simulink model "PII_speed"  (Simulink 7.5)
settings: Solver=ode1  SolverMode=SingleTasking  StartTime=0.0  StopTime=Inf  FixedStep=ts  RelTol=1e-3
PostLoadFcn:
  | , if any(exist('dsrtsu_mdlpostloadfcn', 'file') == [2, 3, 6]), try dsrtsu_mdlpostloadfcn('Execute', bdroot); catch fprintf('Error in PostLoadFcn (dsrtsu_mdlpostloadfcn) for model "%s":\n %s\n', bdroot, lasterr); end, end,
values from neighbouring files (symbols this model uses):
  Amp = 0    [RUN.m]
  en = 0    [RUN.m]
  f = 0.20    (= 0.2)    [RUN.m]
  g = 1    [RUN.m]
  kii = 660    [RUN.m]
  kpi = 2.0    (= 2)    [RUN.m]
  limit = 1    [RUN.m]
  nap = 0    [RUN.m]
  obc_del = 0.7    [RUN.m]
  obc_del2 = 1.3    [RUN.m]
  obc_en = 0    [RUN.m]
  obc_en1 = 0    [RUN.m]
  offset = 0    [RUN.m]
  res = 1    [RUN.m]
  res1 = 1    [RUN.m]
  start = 0    [RUN.m]
  Tf = 0.01    [RUN.m]
  Ts_i = 0.0002    [RUN.m]
  Ts_w = 0.001    [RUN.m]
undefined symbols (not defined in the file or in its folder): k1_singletons, k1k, k2_singletons, k2k, k3_singletons, k3k, kdu, Ki_singletons, Kik, ku, mf
libraries: fuzblock x15, rtilib1103 x6, simulink_extras x1
(part 2 of 2)

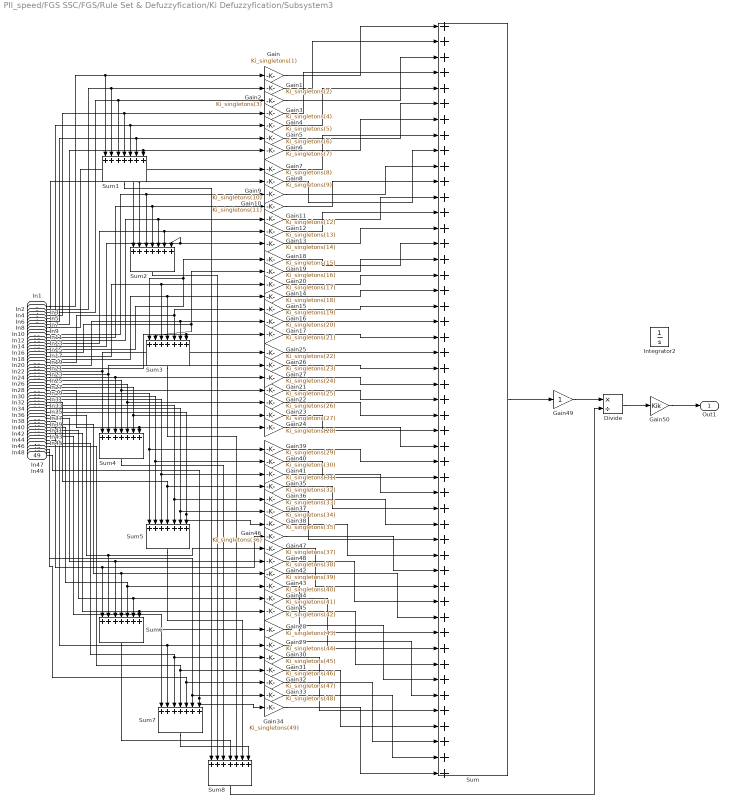
== system PII_speed/FGS SSC/FGS/Rule Set & Defuzzyfication/Ki Defuzzyfication/Subsystem3 ==
  In1 : Inport
  In2 : Inport  Port=2
  In3 : Inport  Port=3
  In4 : Inport  Port=4
  In5 : Inport  Port=5
  In6 : Inport  Port=6
  In7 : Inport  Port=7
  In8 : Inport  Port=8
  In9 : Inport  Port=9
  In10 : Inport  Port=10
  In11 : Inport  Port=11
  In12 : Inport  Port=12
  In13 : Inport  Port=13
  In14 : Inport  Port=14
  In15 : Inport  Port=15
  In16 : Inport  Port=16
  In17 : Inport  Port=17
  In18 : Inport  Port=18
  In19 : Inport  Port=19
  In20 : Inport  Port=20
  In21 : Inport  Port=21
  In22 : Inport  Port=22
  In23 : Inport  Port=23
  In24 : Inport  Port=24
  In25 : Inport  Port=25
  In26 : Inport  Port=26
  In27 : Inport  Port=27
  In28 : Inport  Port=28
  In29 : Inport  Port=29
  In30 : Inport  Port=30
  In31 : Inport  Port=31
  In32 : Inport  Port=32
  In33 : Inport  Port=33
  In34 : Inport  Port=34
  In35 : Inport  Port=35
  In36 : Inport  Port=36
  In37 : Inport  Port=37
  In38 : Inport  Port=38
  In39 : Inport  Port=39
  In40 : Inport  Port=40
  In41 : Inport  Port=41
  In42 : Inport  Port=42
  In43 : Inport  Port=43
  In44 : Inport  Port=44
  In45 : Inport  Port=45
  In46 : Inport  Port=46
  In47 : Inport  Port=47
  In48 : Inport  Port=48
  In49 : Inport  Port=49
  Divide : Product  Inputs=*/
  Gain : Gain  Gain=Ki_singletons(1)
  Gain1 : Gain  Gain=Ki_singletons(2)
  Gain10 : Gain  Gain=Ki_singletons(11)
  Gain11 : Gain  Gain=Ki_singletons(12)
  Gain12 : Gain  Gain=Ki_singletons(13)
  Gain13 : Gain  Gain=Ki_singletons(14)
  Gain14 : Gain  Gain=Ki_singletons(18)
  Gain15 : Gain  Gain=Ki_singletons(19)
  Gain16 : Gain  Gain=Ki_singletons(20)
  Gain17 : Gain  Gain=Ki_singletons(21)
  Gain18 : Gain  Gain=Ki_singletons(15)
  Gain19 : Gain  Gain=Ki_singletons(16)
  Gain2 : Gain  Gain=Ki_singletons(3)
  Gain20 : Gain  Gain=Ki_singletons(17)
  Gain21 : Gain  Gain=Ki_singletons(25)
  Gain22 : Gain  Gain=Ki_singletons(26)
  Gain23 : Gain  Gain=Ki_singletons(27)
  Gain24 : Gain  Gain=Ki_singletons(28)
  Gain25 : Gain  Gain=Ki_singletons(22)
  Gain26 : Gain  Gain=Ki_singletons(23)
  Gain27 : Gain  Gain=Ki_singletons(24)
  Gain28 : Gain  Gain=Ki_singletons(43)
  Gain29 : Gain  Gain=Ki_singletons(44)
  Gain3 : Gain  Gain=Ki_singletons(4)
  Gain30 : Gain  Gain=Ki_singletons(45)
  Gain31 : Gain  Gain=Ki_singletons(46)
  Gain32 : Gain  Gain=Ki_singletons(47)
  Gain33 : Gain  Gain=Ki_singletons(48)
  Gain34 : Gain  Gain=Ki_singletons(49)
  Gain35 : Gain  Gain=Ki_singletons(32)
  Gain36 : Gain  Gain=Ki_singletons(33)
  Gain37 : Gain  Gain=Ki_singletons(34)
  Gain38 : Gain  Gain=Ki_singletons(35)
  Gain39 : Gain  Gain=Ki_singletons(29)
  Gain4 : Gain  Gain=Ki_singletons(5)
  Gain40 : Gain  Gain=Ki_singletons(30)
  Gain41 : Gain  Gain=Ki_singletons(31)
  Gain42 : Gain  Gain=Ki_singletons(39)
  Gain43 : Gain  Gain=Ki_singletons(40)
  Gain44 : Gain  Gain=Ki_singletons(41)
  Gain45 : Gain  Gain=Ki_singletons(42)
  Gain46 : Gain  Gain=Ki_singletons(36)
  Gain47 : Gain  Gain=Ki_singletons(37)
  Gain48 : Gain  Gain=Ki_singletons(38)
  Gain49 : Gain
  Gain5 : Gain  Gain=Ki_singletons(6)
  Gain50 : Gain  Gain=Kik
  Gain6 : Gain  Gain=Ki_singletons(7)
  Gain7 : Gain  Gain=Ki_singletons(8)
  Gain8 : Gain  Gain=Ki_singletons(9)
  Gain9 : Gain  Gain=Ki_singletons(10)
  Integrator2 : Integrator
  Sum : Sum  Inputs=49
  Sum{1..8} (8 alike) : Sum  Inputs=7
  Out1 : Outport
  wires:
  Gain49/1 -> Divide/1
  In4/1 -> Sum1/4, Gain3/1
  Gain25/1 -> Sum/22
  Gain/1 -> Sum/1
  Gain34/1 -> Sum/49
  Gain39/1 -> Sum/29
  Gain13/1 -> Sum/14
  Gain17/1 -> Sum/21
  Gain19/1 -> Sum/16
  Gain12/1 -> Sum/13
  Gain40/1 -> Sum/30
  Gain35/1 -> Sum/32
  Gain9/1 -> Sum/10
  Gain6/1 -> Sum/7
  Gain27/1 -> Sum/24
  Gain11/1 -> Sum/12
  Gain15/1 -> Sum/19
  Gain10/1 -> Sum/11
  Gain22/1 -> Sum/26
  Gain23/1 -> Sum/27
  Gain8/1 -> Sum/9
  Gain38/1 -> Sum/35
  Gain46/1 -> Sum/36
  Gain37/1 -> Sum/34
  Gain16/1 -> Sum/20
  Gain36/1 -> Sum/33
  Gain18/1 -> Sum/15
  Gain14/1 -> Sum/18
  Gain5/1 -> Sum/6
  Gain47/1 -> Sum/37
  Gain26/1 -> Sum/23
  Gain4/1 -> Sum/5
  Gain7/1 -> Sum/8
  Gain20/1 -> Sum/17
  Gain41/1 -> Sum/31
  Gain21/1 -> Sum/25
  Gain24/1 -> Sum/28
  Sum2/1 -> Sum8/2
  Gain33/1 -> Sum/48
  Gain1/1 -> Sum/2
  Sum6/1 -> Sum8/4
  Sum5/1 -> Sum8/6
  Sum4/1 -> Sum8/3
  Sum/1 -> Gain49/1
  Sum8/1 -> Divide/2
  Gain31/1 -> Sum/46
  Gain3/1 -> Sum/4
  Gain44/1 -> Sum/41
  Gain28/1 -> Sum/43
  Gain42/1 -> Sum/39
  Gain2/1 -> Sum/3
  Sum7/1 -> Sum8/7
  Gain29/1 -> Sum/44
  Gain45/1 -> Sum/42
  Gain32/1 -> Sum/47
  Gain30/1 -> Sum/45
  Gain48/1 -> Sum/38
  Gain43/1 -> Sum/40
  Sum1/1 -> Sum8/1
  Sum3/1 -> Sum8/5
  In17/1 -> Sum3/3, Gain20/1
  In20/1 -> Sum3/6, Gain16/1
  In18/1 -> Sum3/4, Gain14/1
  In10/1 -> Sum2/3, Gain9/1
  In14/1 -> Sum2/7, Gain13/1
  In9/1 -> Sum2/2, Gain8/1
  In3/1 -> Sum1/3, Gain2/1
  In15/1 -> Gain18/1, Sum3/1
  In8/1 -> Sum2/1, Gain7/1
  In38/1 -> Gain46/1, Sum6/1
  In37/1 -> Gain48/1, Sum6/3
  In24/1 -> Sum4/3, Gain27/1
  In31/1 -> Gain41/1, Sum5/3
  In22/1 -> Gain25/1, Sum4/1
  In21/1 -> Sum3/7, Gain17/1
  In34/1 -> Gain37/1, Sum5/6
  In19/1 -> Gain15/1, Sum3/5
  In26/1 -> Sum4/5, Gain22/1
  In41/1 -> Gain44/1, Sum6/6
  In43/1 -> Gain28/1, Sum7/1
  In11/1 -> Sum2/4, Gain10/1
  In16/1 -> Gain19/1, Sum3/2
  In25/1 -> Sum4/4, Gain21/1
  In28/1 -> Sum4/7, Gain24/1
  In35/1 -> Gain38/1, Sum5/7
  In12/1 -> Sum2/5, Gain11/1
  In13/1 -> Sum2/6, Gain12/1
  In40/1 -> Gain43/1, Sum6/5
  In33/1 -> Gain36/1, Sum5/5
  In29/1 -> Gain39/1, Sum5/1
  In23/1 -> Gain26/1, Sum4/2
  In36/1 -> Gain47/1, Sum6/2
  In27/1 -> Sum4/6, Gain23/1
  In32/1 -> Gain35/1, Sum5/4
  In30/1 -> Gain40/1, Sum5/2
  In42/1 -> Gain45/1, Sum6/7
  In49/1 -> Gain34/1, Sum7/7
  In44/1 -> Sum7/2, Gain29/1
  In39/1 -> Gain42/1, Sum6/4
  In6/1 -> Sum1/6, Gain5/1
  In46/1 -> Gain31/1, Sum7/4
  In2/1 -> Sum1/2, Gain1/1
  In47/1 -> Gain32/1, Sum7/5
  In5/1 -> Sum1/5, Gain4/1
  In45/1 -> Gain30/1, Sum7/3
  In7/1 -> Sum1/7, Gain6/1
  In1/1 -> Sum1/1, Gain/1
  In48/1 -> Gain33/1, Sum7/6
  Divide/1 -> Gain50/1
  Gain50/1 -> Out1/1

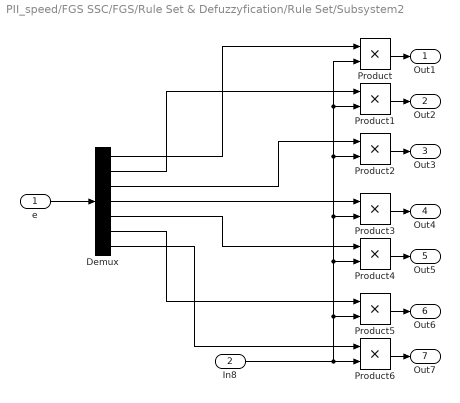
== system PII_speed/FGS SSC/FGS/Rule Set & Defuzzyfication/Rule Set/Subsystem2 ==
  e : Inport
  In8 : Inport  Port=2
  Demux : Demux  Outputs=7
  Product{,1..6} (7 alike) : Product
  Out1 : Outport
  Out2 : Outport  Port=2
  Out3 : Outport  Port=3
  Out4 : Outport  Port=4
  Out5 : Outport  Port=5
  Out6 : Outport  Port=6
  Out7 : Outport  Port=7
  wires:
  Product2/1 -> Out3/1
  Product5/1 -> Out6/1
  Product6/1 -> Out7/1
  Product3/1 -> Out4/1
  Product1/1 -> Out2/1
  Product4/1 -> Out5/1
  Product/1 -> Out1/1
  In8/1 -> Product6/2, Product/2, Product1/2, Product2/2, Product3/2, Product4/2, Product5/2
  e/1 -> Demux/1
  Demux/1 -> Product/1
  Demux/2 -> Product1/1
  Demux/3 -> Product2/1
  Demux/4 -> Product3/1
  Demux/5 -> Product4/1
  Demux/6 -> Product5/1
  Demux/7 -> Product6/1

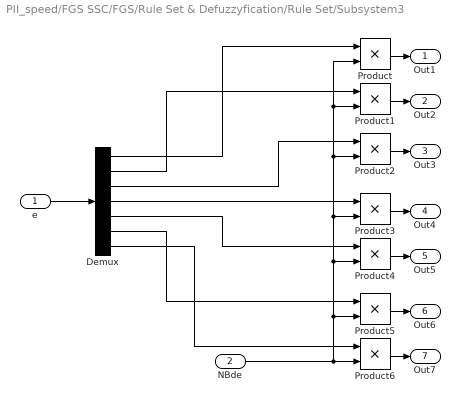
== system PII_speed/FGS SSC/FGS/Rule Set & Defuzzyfication/Rule Set/Subsystem3 ==
  e : Inport
  NBde : Inport  Port=2
  Demux : Demux  Outputs=7
  Product{,1..6} (7 alike) : Product
  Out1 : Outport
  Out2 : Outport  Port=2
  Out3 : Outport  Port=3
  Out4 : Outport  Port=4
  Out5 : Outport  Port=5
  Out6 : Outport  Port=6
  Out7 : Outport  Port=7
  wires:
  Demux/7 -> Product6/1
  Demux/6 -> Product5/1
  Demux/5 -> Product4/1
  Demux/4 -> Product3/1
  Demux/3 -> Product2/1
  Demux/2 -> Product1/1
  Demux/1 -> Product/1
  e/1 -> Demux/1
  NBde/1 -> Product5/2, Product4/2, Product3/2, Product2/2, Product1/2, Product/2, Product6/2
  Product/1 -> Out1/1
  Product4/1 -> Out5/1
  Product1/1 -> Out2/1
  Product3/1 -> Out4/1
  Product6/1 -> Out7/1
  Product5/1 -> Out6/1
  Product2/1 -> Out3/1

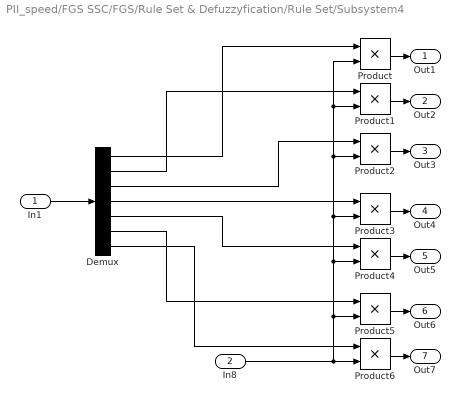
== system PII_speed/FGS SSC/FGS/Rule Set & Defuzzyfication/Rule Set/Subsystem4 ==
  In1 : Inport
  In8 : Inport  Port=2
  Demux : Demux  Outputs=7
  Product{,1..6} (7 alike) : Product
  Out1 : Outport
  Out2 : Outport  Port=2
  Out3 : Outport  Port=3
  Out4 : Outport  Port=4
  Out5 : Outport  Port=5
  Out6 : Outport  Port=6
  Out7 : Outport  Port=7
  wires:
  Demux/7 -> Product6/1
  Demux/6 -> Product5/1
  Demux/5 -> Product4/1
  Demux/4 -> Product3/1
  Demux/3 -> Product2/1
  Demux/2 -> Product1/1
  Demux/1 -> Product/1
  In1/1 -> Demux/1
  In8/1 -> Product5/2, Product4/2, Product3/2, Product2/2, Product1/2, Product/2, Product6/2
  Product/1 -> Out1/1
  Product4/1 -> Out5/1
  Product1/1 -> Out2/1
  Product3/1 -> Out4/1
  Product6/1 -> Out7/1
  Product5/1 -> Out6/1
  Product2/1 -> Out3/1

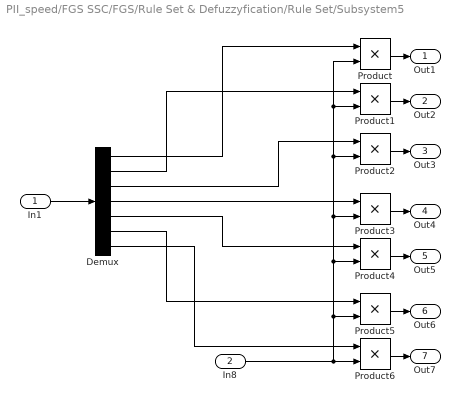
== system PII_speed/FGS SSC/FGS/Rule Set & Defuzzyfication/Rule Set/Subsystem5 ==
  In1 : Inport
  In8 : Inport  Port=2
  Demux : Demux  Outputs=7
  Product{,1..6} (7 alike) : Product
  Out1 : Outport
  Out2 : Outport  Port=2
  Out3 : Outport  Port=3
  Out4 : Outport  Port=4
  Out5 : Outport  Port=5
  Out6 : Outport  Port=6
  Out7 : Outport  Port=7
  wires:
  Demux/7 -> Product6/1
  Demux/6 -> Product5/1
  Demux/5 -> Product4/1
  Demux/4 -> Product3/1
  Demux/3 -> Product2/1
  Demux/2 -> Product1/1
  Demux/1 -> Product/1
  In1/1 -> Demux/1
  In8/1 -> Product5/2, Product4/2, Product3/2, Product2/2, Product1/2, Product/2, Product6/2
  Product/1 -> Out1/1
  Product4/1 -> Out5/1
  Product1/1 -> Out2/1
  Product3/1 -> Out4/1
  Product6/1 -> Out7/1
  Product5/1 -> Out6/1
  Product2/1 -> Out3/1

== system PII_speed/FGS SSC/FGS/Rule Set & Defuzzyfication/Rule Set/Subsystem6 ==
  In1 : Inport
  In8 : Inport  Port=2
  Demux : Demux  Outputs=7
  Product{,1..6} (7 alike) : Product
  Out1 : Outport
  Out2 : Outport  Port=2
  Out3 : Outport  Port=3
  Out4 : Outport  Port=4
  Out5 : Outport  Port=5
  Out6 : Outport  Port=6
  Out7 : Outport  Port=7
  wires:
  Product2/1 -> Out3/1
  Product5/1 -> Out6/1
  Product6/1 -> Out7/1
  Product3/1 -> Out4/1
  Product1/1 -> Out2/1
  Product4/1 -> Out5/1
  Product/1 -> Out1/1
  In8/1 -> Product6/2, Product/2, Product1/2, Product2/2, Product3/2, Product4/2, Product5/2
  In1/1 -> Demux/1
  Demux/1 -> Product/1
  Demux/2 -> Product1/1
  Demux/3 -> Product2/1
  Demux/4 -> Product3/1
  Demux/5 -> Product4/1
  Demux/6 -> Product5/1
  Demux/7 -> Product6/1

== system PII_speed/FGS SSC/FGS/Rule Set & Defuzzyfication/Rule Set/Subsystem7 ==
  In1 : Inport
  In8 : Inport  Port=2
  Demux : Demux  Outputs=7
  Product{,1..6} (7 alike) : Product
  Out1 : Outport
  Out2 : Outport  Port=2
  Out3 : Outport  Port=3
  Out4 : Outport  Port=4
  Out5 : Outport  Port=5
  Out6 : Outport  Port=6
  Out7 : Outport  Port=7
  wires:
  Product2/1 -> Out3/1
  Product5/1 -> Out6/1
  Product6/1 -> Out7/1
  Product3/1 -> Out4/1
  Product1/1 -> Out2/1
  Product4/1 -> Out5/1
  Product/1 -> Out1/1
  In8/1 -> Product6/2, Product/2, Product1/2, Product2/2, Product3/2, Product4/2, Product5/2
  In1/1 -> Demux/1
  Demux/1 -> Product/1
  Demux/2 -> Product1/1
  Demux/3 -> Product2/1
  Demux/4 -> Product3/1
  Demux/5 -> Product4/1
  Demux/6 -> Product5/1
  Demux/7 -> Product6/1

== system PII_speed/FGS SSC/FGS/Rule Set & Defuzzyfication/Rule Set/Subsystem8 ==
  In1 : Inport
  In8 : Inport  Port=2
  Demux : Demux  Outputs=7
  Product{,1..6} (7 alike) : Product
  Out1 : Outport
  Out2 : Outport  Port=2
  Out3 : Outport  Port=3
  Out4 : Outport  Port=4
  Out5 : Outport  Port=5
  Out6 : Outport  Port=6
  Out7 : Outport  Port=7
  wires:
  Demux/7 -> Product6/1
  Demux/6 -> Product5/1
  Demux/5 -> Product4/1
  Demux/4 -> Product3/1
  Demux/3 -> Product2/1
  Demux/2 -> Product1/1
  Demux/1 -> Product/1
  In1/1 -> Demux/1
  In8/1 -> Product5/2, Product4/2, Product3/2, Product2/2, Product1/2, Product/2, Product6/2
  Product/1 -> Out1/1
  Product4/1 -> Out5/1
  Product1/1 -> Out2/1
  Product3/1 -> Out4/1
  Product6/1 -> Out7/1
  Product5/1 -> Out6/1
  Product2/1 -> Out3/1

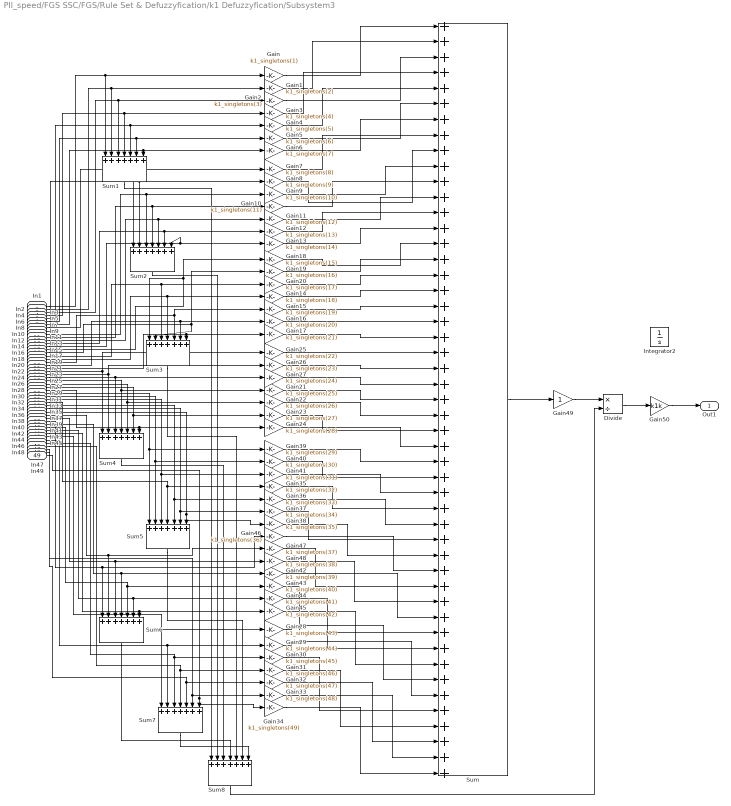
== system PII_speed/FGS SSC/FGS/Rule Set & Defuzzyfication/k1 Defuzzyfication/Subsystem3 ==
  In1 : Inport
  In2 : Inport  Port=2
  In3 : Inport  Port=3
  In4 : Inport  Port=4
  In5 : Inport  Port=5
  In6 : Inport  Port=6
  In7 : Inport  Port=7
  In8 : Inport  Port=8
  In9 : Inport  Port=9
  In10 : Inport  Port=10
  In11 : Inport  Port=11
  In12 : Inport  Port=12
  In13 : Inport  Port=13
  In14 : Inport  Port=14
  In15 : Inport  Port=15
  In16 : Inport  Port=16
  In17 : Inport  Port=17
  In18 : Inport  Port=18
  In19 : Inport  Port=19
  In20 : Inport  Port=20
  In21 : Inport  Port=21
  In22 : Inport  Port=22
  In23 : Inport  Port=23
  In24 : Inport  Port=24
  In25 : Inport  Port=25
  In26 : Inport  Port=26
  In27 : Inport  Port=27
  In28 : Inport  Port=28
  In29 : Inport  Port=29
  In30 : Inport  Port=30
  In31 : Inport  Port=31
  In32 : Inport  Port=32
  In33 : Inport  Port=33
  In34 : Inport  Port=34
  In35 : Inport  Port=35
  In36 : Inport  Port=36
  In37 : Inport  Port=37
  In38 : Inport  Port=38
  In39 : Inport  Port=39
  In40 : Inport  Port=40
  In41 : Inport  Port=41
  In42 : Inport  Port=42
  In43 : Inport  Port=43
  In44 : Inport  Port=44
  In45 : Inport  Port=45
  In46 : Inport  Port=46
  In47 : Inport  Port=47
  In48 : Inport  Port=48
  In49 : Inport  Port=49
  Divide : Product  Inputs=*/
  Gain : Gain  Gain=k1_singletons(1)
  Gain1 : Gain  Gain=k1_singletons(2)
  Gain10 : Gain  Gain=k1_singletons(11)
  Gain11 : Gain  Gain=k1_singletons(12)
  Gain12 : Gain  Gain=k1_singletons(13)
  Gain13 : Gain  Gain=k1_singletons(14)
  Gain14 : Gain  Gain=k1_singletons(18)
  Gain15 : Gain  Gain=k1_singletons(19)
  Gain16 : Gain  Gain=k1_singletons(20)
  Gain17 : Gain  Gain=k1_singletons(21)
  Gain18 : Gain  Gain=k1_singletons(15)
  Gain19 : Gain  Gain=k1_singletons(16)
  Gain2 : Gain  Gain=k1_singletons(3)
  Gain20 : Gain  Gain=k1_singletons(17)
  Gain21 : Gain  Gain=k1_singletons(25)
  Gain22 : Gain  Gain=k1_singletons(26)
  Gain23 : Gain  Gain=k1_singletons(27)
  Gain24 : Gain  Gain=k1_singletons(28)
  Gain25 : Gain  Gain=k1_singletons(22)
  Gain26 : Gain  Gain=k1_singletons(23)
  Gain27 : Gain  Gain=k1_singletons(24)
  Gain28 : Gain  Gain=k1_singletons(43)
  Gain29 : Gain  Gain=k1_singletons(44)
  Gain3 : Gain  Gain=k1_singletons(4)
  Gain30 : Gain  Gain=k1_singletons(45)
  Gain31 : Gain  Gain=k1_singletons(46)
  Gain32 : Gain  Gain=k1_singletons(47)
  Gain33 : Gain  Gain=k1_singletons(48)
  Gain34 : Gain  Gain=k1_singletons(49)
  Gain35 : Gain  Gain=k1_singletons(32)
  Gain36 : Gain  Gain=k1_singletons(33)
  Gain37 : Gain  Gain=k1_singletons(34)
  Gain38 : Gain  Gain=k1_singletons(35)
  Gain39 : Gain  Gain=k1_singletons(29)
  Gain4 : Gain  Gain=k1_singletons(5)
  Gain40 : Gain  Gain=k1_singletons(30)
  Gain41 : Gain  Gain=k1_singletons(31)
  Gain42 : Gain  Gain=k1_singletons(39)
  Gain43 : Gain  Gain=k1_singletons(40)
  Gain44 : Gain  Gain=k1_singletons(41)
  Gain45 : Gain  Gain=k1_singletons(42)
  Gain46 : Gain  Gain=k1_singletons(36)
  Gain47 : Gain  Gain=k1_singletons(37)
  Gain48 : Gain  Gain=k1_singletons(38)
  Gain49 : Gain
  Gain5 : Gain  Gain=k1_singletons(6)
  Gain50 : Gain  Gain=k1k
  Gain6 : Gain  Gain=k1_singletons(7)
  Gain7 : Gain  Gain=k1_singletons(8)
  Gain8 : Gain  Gain=k1_singletons(9)
  Gain9 : Gain  Gain=k1_singletons(10)
  Integrator2 : Integrator
  Sum : Sum  Inputs=49
  Sum{1..8} (8 alike) : Sum  Inputs=7
  Out1 : Outport
  wires:
  Gain50/1 -> Out1/1
  Divide/1 -> Gain50/1
  In48/1 -> Sum7/6, Gain33/1
  In1/1 -> Gain/1, Sum1/1
  In7/1 -> Gain6/1, Sum1/7
  In45/1 -> Sum7/3, Gain30/1
  In5/1 -> Gain4/1, Sum1/5
  In47/1 -> Sum7/5, Gain32/1
  In2/1 -> Gain1/1, Sum1/2
  In46/1 -> Sum7/4, Gain31/1
  In6/1 -> Gain5/1, Sum1/6
  In39/1 -> Sum6/4, Gain42/1
  In44/1 -> Gain29/1, Sum7/2
  In49/1 -> Sum7/7, Gain34/1
  In42/1 -> Sum6/7, Gain45/1
  In30/1 -> Sum5/2, Gain40/1
  In32/1 -> Sum5/4, Gain35/1
  In27/1 -> Gain23/1, Sum4/6
  In36/1 -> Sum6/2, Gain47/1
  In23/1 -> Sum4/2, Gain26/1
  In29/1 -> Sum5/1, Gain39/1
  In33/1 -> Sum5/5, Gain36/1
  In40/1 -> Sum6/5, Gain43/1
  In13/1 -> Gain12/1, Sum2/6
  In12/1 -> Gain11/1, Sum2/5
  In35/1 -> Sum5/7, Gain38/1
  In28/1 -> Gain24/1, Sum4/7
  In25/1 -> Gain21/1, Sum4/4
  In16/1 -> Sum3/2, Gain19/1
  In11/1 -> Gain10/1, Sum2/4
  In43/1 -> Sum7/1, Gain28/1
  In41/1 -> Sum6/6, Gain44/1
  In26/1 -> Gain22/1, Sum4/5
  In19/1 -> Sum3/5, Gain15/1
  In34/1 -> Sum5/6, Gain37/1
  In21/1 -> Gain17/1, Sum3/7
  In22/1 -> Sum4/1, Gain25/1
  In31/1 -> Sum5/3, Gain41/1
  In24/1 -> Gain27/1, Sum4/3
  In37/1 -> Sum6/3, Gain48/1
  In38/1 -> Sum6/1, Gain46/1
  In8/1 -> Gain7/1, Sum2/1
  In15/1 -> Sum3/1, Gain18/1
  In3/1 -> Gain2/1, Sum1/3
  In9/1 -> Gain8/1, Sum2/2
  In14/1 -> Gain13/1, Sum2/7
  In10/1 -> Gain9/1, Sum2/3
  In18/1 -> Gain14/1, Sum3/4
  In20/1 -> Gain16/1, Sum3/6
  In17/1 -> Gain20/1, Sum3/3
  Sum3/1 -> Sum8/5
  Sum1/1 -> Sum8/1
  Gain43/1 -> Sum/40
  Gain48/1 -> Sum/38
  Gain30/1 -> Sum/45
  Gain32/1 -> Sum/47
  Gain45/1 -> Sum/42
  Gain29/1 -> Sum/44
  Sum7/1 -> Sum8/7
  Gain2/1 -> Sum/3
  Gain42/1 -> Sum/39
  Gain28/1 -> Sum/43
  Gain44/1 -> Sum/41
  Gain3/1 -> Sum/4
  Gain31/1 -> Sum/46
  Sum8/1 -> Divide/2
  Sum/1 -> Gain49/1
  Sum4/1 -> Sum8/3
  Sum5/1 -> Sum8/6
  Sum6/1 -> Sum8/4
  Gain1/1 -> Sum/2
  Gain33/1 -> Sum/48
  Sum2/1 -> Sum8/2
  Gain24/1 -> Sum/28
  Gain21/1 -> Sum/25
  Gain41/1 -> Sum/31
  Gain20/1 -> Sum/17
  Gain7/1 -> Sum/8
  Gain4/1 -> Sum/5
  Gain26/1 -> Sum/23
  Gain47/1 -> Sum/37
  Gain5/1 -> Sum/6
  Gain14/1 -> Sum/18
  Gain18/1 -> Sum/15
  Gain36/1 -> Sum/33
  Gain16/1 -> Sum/20
  Gain37/1 -> Sum/34
  Gain46/1 -> Sum/36
  Gain38/1 -> Sum/35
  Gain8/1 -> Sum/9
  Gain23/1 -> Sum/27
  Gain22/1 -> Sum/26
  Gain10/1 -> Sum/11
  Gain15/1 -> Sum/19
  Gain11/1 -> Sum/12
  Gain27/1 -> Sum/24
  Gain6/1 -> Sum/7
  Gain9/1 -> Sum/10
  Gain35/1 -> Sum/32
  Gain40/1 -> Sum/30
  Gain12/1 -> Sum/13
  Gain19/1 -> Sum/16
  Gain17/1 -> Sum/21
  Gain13/1 -> Sum/14
  Gain39/1 -> Sum/29
  Gain34/1 -> Sum/49
  Gain/1 -> Sum/1
  Gain25/1 -> Sum/22
  In4/1 -> Gain3/1, Sum1/4
  Gain49/1 -> Divide/1

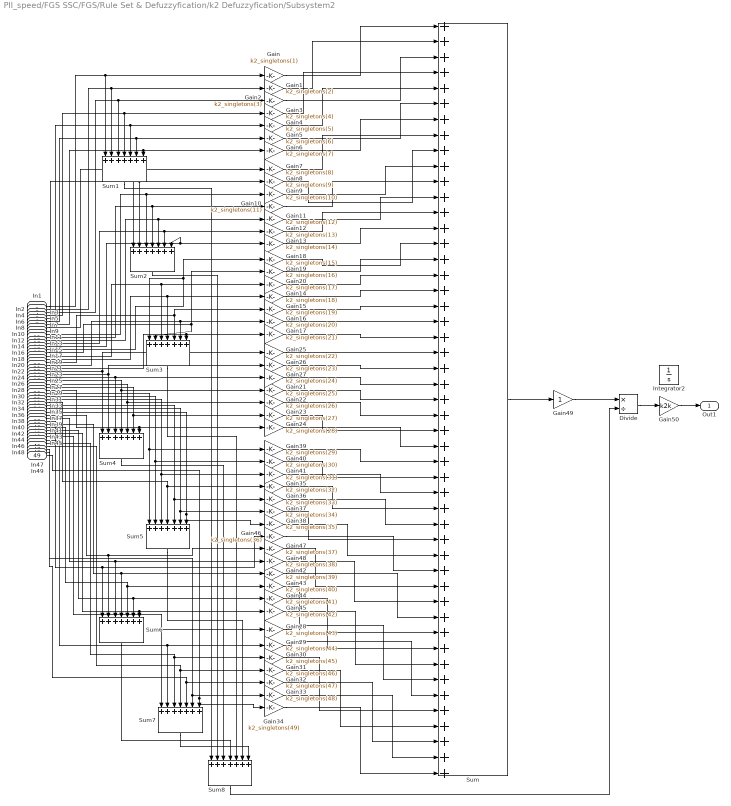
== system PII_speed/FGS SSC/FGS/Rule Set & Defuzzyfication/k2 Defuzzyfication/Subsystem2 ==
  In1 : Inport
  In2 : Inport  Port=2
  In3 : Inport  Port=3
  In4 : Inport  Port=4
  In5 : Inport  Port=5
  In6 : Inport  Port=6
  In7 : Inport  Port=7
  In8 : Inport  Port=8
  In9 : Inport  Port=9
  In10 : Inport  Port=10
  In11 : Inport  Port=11
  In12 : Inport  Port=12
  In13 : Inport  Port=13
  In14 : Inport  Port=14
  In15 : Inport  Port=15
  In16 : Inport  Port=16
  In17 : Inport  Port=17
  In18 : Inport  Port=18
  In19 : Inport  Port=19
  In20 : Inport  Port=20
  In21 : Inport  Port=21
  In22 : Inport  Port=22
  In23 : Inport  Port=23
  In24 : Inport  Port=24
  In25 : Inport  Port=25
  In26 : Inport  Port=26
  In27 : Inport  Port=27
  In28 : Inport  Port=28
  In29 : Inport  Port=29
  In30 : Inport  Port=30
  In31 : Inport  Port=31
  In32 : Inport  Port=32
  In33 : Inport  Port=33
  In34 : Inport  Port=34
  In35 : Inport  Port=35
  In36 : Inport  Port=36
  In37 : Inport  Port=37
  In38 : Inport  Port=38
  In39 : Inport  Port=39
  In40 : Inport  Port=40
  In41 : Inport  Port=41
  In42 : Inport  Port=42
  In43 : Inport  Port=43
  In44 : Inport  Port=44
  In45 : Inport  Port=45
  In46 : Inport  Port=46
  In47 : Inport  Port=47
  In48 : Inport  Port=48
  In49 : Inport  Port=49
  Divide : Product  Inputs=*/
  Gain : Gain  Gain=k2_singletons(1)
  Gain1 : Gain  Gain=k2_singletons(2)
  Gain10 : Gain  Gain=k2_singletons(11)
  Gain11 : Gain  Gain=k2_singletons(12)
  Gain12 : Gain  Gain=k2_singletons(13)
  Gain13 : Gain  Gain=k2_singletons(14)
  Gain14 : Gain  Gain=k2_singletons(18)
  Gain15 : Gain  Gain=k2_singletons(19)
  Gain16 : Gain  Gain=k2_singletons(20)
  Gain17 : Gain  Gain=k2_singletons(21)
  Gain18 : Gain  Gain=k2_singletons(15)
  Gain19 : Gain  Gain=k2_singletons(16)
  Gain2 : Gain  Gain=k2_singletons(3)
  Gain20 : Gain  Gain=k2_singletons(17)
  Gain21 : Gain  Gain=k2_singletons(25)
  Gain22 : Gain  Gain=k2_singletons(26)
  Gain23 : Gain  Gain=k2_singletons(27)
  Gain24 : Gain  Gain=k2_singletons(28)
  Gain25 : Gain  Gain=k2_singletons(22)
  Gain26 : Gain  Gain=k2_singletons(23)
  Gain27 : Gain  Gain=k2_singletons(24)
  Gain28 : Gain  Gain=k2_singletons(43)
  Gain29 : Gain  Gain=k2_singletons(44)
  Gain3 : Gain  Gain=k2_singletons(4)
  Gain30 : Gain  Gain=k2_singletons(45)
  Gain31 : Gain  Gain=k2_singletons(46)
  Gain32 : Gain  Gain=k2_singletons(47)
  Gain33 : Gain  Gain=k2_singletons(48)
  Gain34 : Gain  Gain=k2_singletons(49)
  Gain35 : Gain  Gain=k2_singletons(32)
  Gain36 : Gain  Gain=k2_singletons(33)
  Gain37 : Gain  Gain=k2_singletons(34)
  Gain38 : Gain  Gain=k2_singletons(35)
  Gain39 : Gain  Gain=k2_singletons(29)
  Gain4 : Gain  Gain=k2_singletons(5)
  Gain40 : Gain  Gain=k2_singletons(30)
  Gain41 : Gain  Gain=k2_singletons(31)
  Gain42 : Gain  Gain=k2_singletons(39)
  Gain43 : Gain  Gain=k2_singletons(40)
  Gain44 : Gain  Gain=k2_singletons(41)
  Gain45 : Gain  Gain=k2_singletons(42)
  Gain46 : Gain  Gain=k2_singletons(36)
  Gain47 : Gain  Gain=k2_singletons(37)
  Gain48 : Gain  Gain=k2_singletons(38)
  Gain49 : Gain
  Gain5 : Gain  Gain=k2_singletons(6)
  Gain50 : Gain  Gain=k2k
  Gain6 : Gain  Gain=k2_singletons(7)
  Gain7 : Gain  Gain=k2_singletons(8)
  Gain8 : Gain  Gain=k2_singletons(9)
  Gain9 : Gain  Gain=k2_singletons(10)
  Integrator2 : Integrator
  Sum : Sum  Inputs=49
  Sum{1..8} (8 alike) : Sum  Inputs=7
  Out1 : Outport
  wires:
  Gain49/1 -> Divide/1
  In4/1 -> Sum1/4, Gain3/1
  Gain25/1 -> Sum/22
  Gain/1 -> Sum/1
  Gain34/1 -> Sum/49
  Gain39/1 -> Sum/29
  Gain13/1 -> Sum/14
  Gain17/1 -> Sum/21
  Gain19/1 -> Sum/16
  Gain12/1 -> Sum/13
  Gain40/1 -> Sum/30
  Gain35/1 -> Sum/32
  Gain9/1 -> Sum/10
  Gain6/1 -> Sum/7
  Gain27/1 -> Sum/24
  Gain11/1 -> Sum/12
  Gain15/1 -> Sum/19
  Gain10/1 -> Sum/11
  Gain22/1 -> Sum/26
  Gain23/1 -> Sum/27
  Gain8/1 -> Sum/9
  Gain38/1 -> Sum/35
  Gain46/1 -> Sum/36
  Gain37/1 -> Sum/34
  Gain16/1 -> Sum/20
  Gain36/1 -> Sum/33
  Gain18/1 -> Sum/15
  Gain14/1 -> Sum/18
  Gain5/1 -> Sum/6
  Gain47/1 -> Sum/37
  Gain26/1 -> Sum/23
  Gain4/1 -> Sum/5
  Gain7/1 -> Sum/8
  Gain20/1 -> Sum/17
  Gain41/1 -> Sum/31
  Gain21/1 -> Sum/25
  Gain24/1 -> Sum/28
  Sum2/1 -> Sum8/2
  Gain33/1 -> Sum/48
  Gain1/1 -> Sum/2
  Sum6/1 -> Sum8/4
  Sum5/1 -> Sum8/6
  Sum4/1 -> Sum8/3
  Sum/1 -> Gain49/1
  Sum8/1 -> Divide/2
  Gain31/1 -> Sum/46
  Gain3/1 -> Sum/4
  Gain44/1 -> Sum/41
  Gain28/1 -> Sum/43
  Gain42/1 -> Sum/39
  Gain2/1 -> Sum/3
  Sum7/1 -> Sum8/7
  Gain29/1 -> Sum/44
  Gain45/1 -> Sum/42
  Gain32/1 -> Sum/47
  Gain30/1 -> Sum/45
  Gain48/1 -> Sum/38
  Gain43/1 -> Sum/40
  Sum1/1 -> Sum8/1
  Sum3/1 -> Sum8/5
  In17/1 -> Sum3/3, Gain20/1
  In20/1 -> Sum3/6, Gain16/1
  In18/1 -> Sum3/4, Gain14/1
  In10/1 -> Sum2/3, Gain9/1
  In14/1 -> Sum2/7, Gain13/1
  In9/1 -> Sum2/2, Gain8/1
  In3/1 -> Sum1/3, Gain2/1
  In15/1 -> Gain18/1, Sum3/1
  In8/1 -> Sum2/1, Gain7/1
  In38/1 -> Gain46/1, Sum6/1
  In37/1 -> Gain48/1, Sum6/3
  In24/1 -> Sum4/3, Gain27/1
  In31/1 -> Gain41/1, Sum5/3
  In22/1 -> Gain25/1, Sum4/1
  In21/1 -> Sum3/7, Gain17/1
  In34/1 -> Gain37/1, Sum5/6
  In19/1 -> Gain15/1, Sum3/5
  In26/1 -> Sum4/5, Gain22/1
  In41/1 -> Gain44/1, Sum6/6
  In43/1 -> Gain28/1, Sum7/1
  In11/1 -> Sum2/4, Gain10/1
  In16/1 -> Gain19/1, Sum3/2
  In25/1 -> Sum4/4, Gain21/1
  In28/1 -> Sum4/7, Gain24/1
  In35/1 -> Gain38/1, Sum5/7
  In12/1 -> Sum2/5, Gain11/1
  In13/1 -> Sum2/6, Gain12/1
  In40/1 -> Gain43/1, Sum6/5
  In33/1 -> Gain36/1, Sum5/5
  In29/1 -> Gain39/1, Sum5/1
  In23/1 -> Gain26/1, Sum4/2
  In36/1 -> Gain47/1, Sum6/2
  In27/1 -> Sum4/6, Gain23/1
  In32/1 -> Gain35/1, Sum5/4
  In30/1 -> Gain40/1, Sum5/2
  In42/1 -> Gain45/1, Sum6/7
  In49/1 -> Gain34/1, Sum7/7
  In44/1 -> Sum7/2, Gain29/1
  In39/1 -> Gain42/1, Sum6/4
  In6/1 -> Sum1/6, Gain5/1
  In46/1 -> Gain31/1, Sum7/4
  In2/1 -> Sum1/2, Gain1/1
  In47/1 -> Gain32/1, Sum7/5
  In5/1 -> Sum1/5, Gain4/1
  In45/1 -> Gain30/1, Sum7/3
  In7/1 -> Sum1/7, Gain6/1
  In1/1 -> Sum1/1, Gain/1
  In48/1 -> Gain33/1, Sum7/6
  Divide/1 -> Gain50/1
  Gain50/1 -> Out1/1

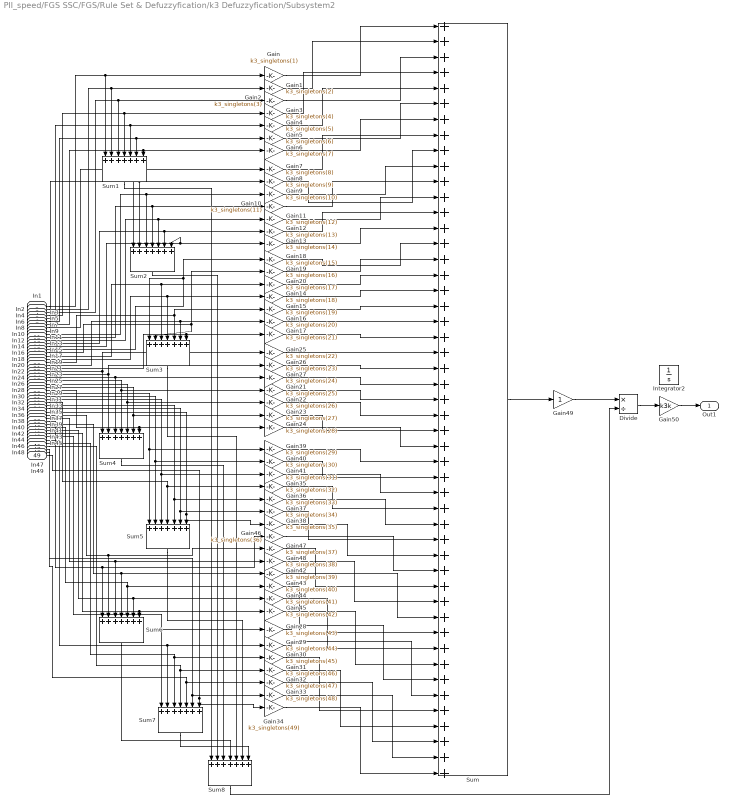
== system PII_speed/FGS SSC/FGS/Rule Set & Defuzzyfication/k3 Defuzzyfication/Subsystem2 ==
  In1 : Inport
  In2 : Inport  Port=2
  In3 : Inport  Port=3
  In4 : Inport  Port=4
  In5 : Inport  Port=5
  In6 : Inport  Port=6
  In7 : Inport  Port=7
  In8 : Inport  Port=8
  In9 : Inport  Port=9
  In10 : Inport  Port=10
  In11 : Inport  Port=11
  In12 : Inport  Port=12
  In13 : Inport  Port=13
  In14 : Inport  Port=14
  In15 : Inport  Port=15
  In16 : Inport  Port=16
  In17 : Inport  Port=17
  In18 : Inport  Port=18
  In19 : Inport  Port=19
  In20 : Inport  Port=20
  In21 : Inport  Port=21
  In22 : Inport  Port=22
  In23 : Inport  Port=23
  In24 : Inport  Port=24
  In25 : Inport  Port=25
  In26 : Inport  Port=26
  In27 : Inport  Port=27
  In28 : Inport  Port=28
  In29 : Inport  Port=29
  In30 : Inport  Port=30
  In31 : Inport  Port=31
  In32 : Inport  Port=32
  In33 : Inport  Port=33
  In34 : Inport  Port=34
  In35 : Inport  Port=35
  In36 : Inport  Port=36
  In37 : Inport  Port=37
  In38 : Inport  Port=38
  In39 : Inport  Port=39
  In40 : Inport  Port=40
  In41 : Inport  Port=41
  In42 : Inport  Port=42
  In43 : Inport  Port=43
  In44 : Inport  Port=44
  In45 : Inport  Port=45
  In46 : Inport  Port=46
  In47 : Inport  Port=47
  In48 : Inport  Port=48
  In49 : Inport  Port=49
  Divide : Product  Inputs=*/
  Gain : Gain  Gain=k3_singletons(1)
  Gain1 : Gain  Gain=k3_singletons(2)
  Gain10 : Gain  Gain=k3_singletons(11)
  Gain11 : Gain  Gain=k3_singletons(12)
  Gain12 : Gain  Gain=k3_singletons(13)
  Gain13 : Gain  Gain=k3_singletons(14)
  Gain14 : Gain  Gain=k3_singletons(18)
  Gain15 : Gain  Gain=k3_singletons(19)
  Gain16 : Gain  Gain=k3_singletons(20)
  Gain17 : Gain  Gain=k3_singletons(21)
  Gain18 : Gain  Gain=k3_singletons(15)
  Gain19 : Gain  Gain=k3_singletons(16)
  Gain2 : Gain  Gain=k3_singletons(3)
  Gain20 : Gain  Gain=k3_singletons(17)
  Gain21 : Gain  Gain=k3_singletons(25)
  Gain22 : Gain  Gain=k3_singletons(26)
  Gain23 : Gain  Gain=k3_singletons(27)
  Gain24 : Gain  Gain=k3_singletons(28)
  Gain25 : Gain  Gain=k3_singletons(22)
  Gain26 : Gain  Gain=k3_singletons(23)
  Gain27 : Gain  Gain=k3_singletons(24)
  Gain28 : Gain  Gain=k3_singletons(43)
  Gain29 : Gain  Gain=k3_singletons(44)
  Gain3 : Gain  Gain=k3_singletons(4)
  Gain30 : Gain  Gain=k3_singletons(45)
  Gain31 : Gain  Gain=k3_singletons(46)
  Gain32 : Gain  Gain=k3_singletons(47)
  Gain33 : Gain  Gain=k3_singletons(48)
  Gain34 : Gain  Gain=k3_singletons(49)
  Gain35 : Gain  Gain=k3_singletons(32)
  Gain36 : Gain  Gain=k3_singletons(33)
  Gain37 : Gain  Gain=k3_singletons(34)
  Gain38 : Gain  Gain=k3_singletons(35)
  Gain39 : Gain  Gain=k3_singletons(29)
  Gain4 : Gain  Gain=k3_singletons(5)
  Gain40 : Gain  Gain=k3_singletons(30)
  Gain41 : Gain  Gain=k3_singletons(31)
  Gain42 : Gain  Gain=k3_singletons(39)
  Gain43 : Gain  Gain=k3_singletons(40)
  Gain44 : Gain  Gain=k3_singletons(41)
  Gain45 : Gain  Gain=k3_singletons(42)
  Gain46 : Gain  Gain=k3_singletons(36)
  Gain47 : Gain  Gain=k3_singletons(37)
  Gain48 : Gain  Gain=k3_singletons(38)
  Gain49 : Gain
  Gain5 : Gain  Gain=k3_singletons(6)
  Gain50 : Gain  Gain=k3k
  Gain6 : Gain  Gain=k3_singletons(7)
  Gain7 : Gain  Gain=k3_singletons(8)
  Gain8 : Gain  Gain=k3_singletons(9)
  Gain9 : Gain  Gain=k3_singletons(10)
  Integrator2 : Integrator
  Sum : Sum  Inputs=49
  Sum{1..8} (8 alike) : Sum  Inputs=7
  Out1 : Outport
  wires:
  Gain50/1 -> Out1/1
  Divide/1 -> Gain50/1
  In48/1 -> Sum7/6, Gain33/1
  In1/1 -> Gain/1, Sum1/1
  In7/1 -> Gain6/1, Sum1/7
  In45/1 -> Sum7/3, Gain30/1
  In5/1 -> Gain4/1, Sum1/5
  In47/1 -> Sum7/5, Gain32/1
  In2/1 -> Gain1/1, Sum1/2
  In46/1 -> Sum7/4, Gain31/1
  In6/1 -> Gain5/1, Sum1/6
  In39/1 -> Sum6/4, Gain42/1
  In44/1 -> Gain29/1, Sum7/2
  In49/1 -> Sum7/7, Gain34/1
  In42/1 -> Sum6/7, Gain45/1
  In30/1 -> Sum5/2, Gain40/1
  In32/1 -> Sum5/4, Gain35/1
  In27/1 -> Gain23/1, Sum4/6
  In36/1 -> Sum6/2, Gain47/1
  In23/1 -> Sum4/2, Gain26/1
  In29/1 -> Sum5/1, Gain39/1
  In33/1 -> Sum5/5, Gain36/1
  In40/1 -> Sum6/5, Gain43/1
  In13/1 -> Gain12/1, Sum2/6
  In12/1 -> Gain11/1, Sum2/5
  In35/1 -> Sum5/7, Gain38/1
  In28/1 -> Gain24/1, Sum4/7
  In25/1 -> Gain21/1, Sum4/4
  In16/1 -> Sum3/2, Gain19/1
  In11/1 -> Gain10/1, Sum2/4
  In43/1 -> Sum7/1, Gain28/1
  In41/1 -> Sum6/6, Gain44/1
  In26/1 -> Gain22/1, Sum4/5
  In19/1 -> Sum3/5, Gain15/1
  In34/1 -> Sum5/6, Gain37/1
  In21/1 -> Gain17/1, Sum3/7
  In22/1 -> Sum4/1, Gain25/1
  In31/1 -> Sum5/3, Gain41/1
  In24/1 -> Gain27/1, Sum4/3
  In37/1 -> Sum6/3, Gain48/1
  In38/1 -> Sum6/1, Gain46/1
  In8/1 -> Gain7/1, Sum2/1
  In15/1 -> Sum3/1, Gain18/1
  In3/1 -> Gain2/1, Sum1/3
  In9/1 -> Gain8/1, Sum2/2
  In14/1 -> Gain13/1, Sum2/7
  In10/1 -> Gain9/1, Sum2/3
  In18/1 -> Gain14/1, Sum3/4
  In20/1 -> Gain16/1, Sum3/6
  In17/1 -> Gain20/1, Sum3/3
  Sum3/1 -> Sum8/5
  Sum1/1 -> Sum8/1
  Gain43/1 -> Sum/40
  Gain48/1 -> Sum/38
  Gain30/1 -> Sum/45
  Gain32/1 -> Sum/47
  Gain45/1 -> Sum/42
  Gain29/1 -> Sum/44
  Sum7/1 -> Sum8/7
  Gain2/1 -> Sum/3
  Gain42/1 -> Sum/39
  Gain28/1 -> Sum/43
  Gain44/1 -> Sum/41
  Gain3/1 -> Sum/4
  Gain31/1 -> Sum/46
  Sum8/1 -> Divide/2
  Sum/1 -> Gain49/1
  Sum4/1 -> Sum8/3
  Sum5/1 -> Sum8/6
  Sum6/1 -> Sum8/4
  Gain1/1 -> Sum/2
  Gain33/1 -> Sum/48
  Sum2/1 -> Sum8/2
  Gain24/1 -> Sum/28
  Gain21/1 -> Sum/25
  Gain41/1 -> Sum/31
  Gain20/1 -> Sum/17
  Gain7/1 -> Sum/8
  Gain4/1 -> Sum/5
  Gain26/1 -> Sum/23
  Gain47/1 -> Sum/37
  Gain5/1 -> Sum/6
  Gain14/1 -> Sum/18
  Gain18/1 -> Sum/15
  Gain36/1 -> Sum/33
  Gain16/1 -> Sum/20
  Gain37/1 -> Sum/34
  Gain46/1 -> Sum/36
  Gain38/1 -> Sum/35
  Gain8/1 -> Sum/9
  Gain23/1 -> Sum/27
  Gain22/1 -> Sum/26
  Gain10/1 -> Sum/11
  Gain15/1 -> Sum/19
  Gain11/1 -> Sum/12
  Gain27/1 -> Sum/24
  Gain6/1 -> Sum/7
  Gain9/1 -> Sum/10
  Gain35/1 -> Sum/32
  Gain40/1 -> Sum/30
  Gain12/1 -> Sum/13
  Gain19/1 -> Sum/16
  Gain17/1 -> Sum/21
  Gain13/1 -> Sum/14
  Gain39/1 -> Sum/29
  Gain34/1 -> Sum/49
  Gain/1 -> Sum/1
  Gain25/1 -> Sum/22
  In4/1 -> Gain3/1, Sum1/4
  Gain49/1 -> Divide/1

== system PII_speed/RTI Data/RTI Data Store/RTI Data Store/RTI Data Store/RTI Data Store ==

== matlab function FGS SSC/FGS/TF calc/MATLAB Function ==
  data: Kif input double; L output double; k1f input double; k2f input double; k3f input double; T2 input double; M output double; Tc input double
function [L,M] = fcn(Kif, k1f, k2f, k3f, T2, Tc)
L = Kif;
M = [(0.203 * T2 * Tc) (k1f * T2 * Tc) (Tc * k2f + T2 + 0.203) (k1f + k3f) Kif];
